simulink subsystem "bodyModel"  (R2026a)
settings: Solver=VariableStepAuto
values from neighbouring files (symbols this model uses):
  aeroParams : value not decoded    [plantParams.sldd]
  vehicleParams = 18.0    [plantParams.sldd]
libraries: matrix_library x1, vrlib x1, simulink_extras x1
settings Model: DataDictionary=plantParams.sldd  EnableAccessToBaseWorkspace=off  Creator=maxhu  LastModifiedBy=maxhu

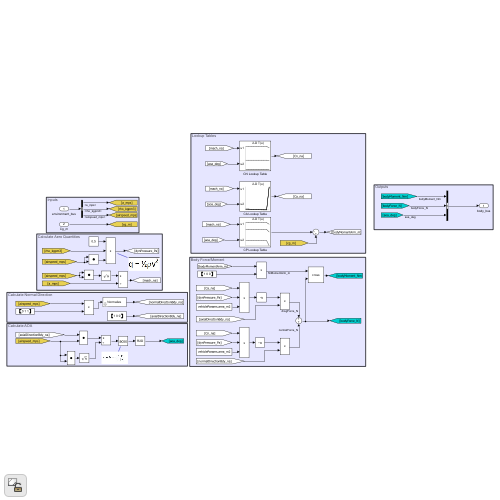
[thumbnail: Simulink's stored preview of the top-level diagram]
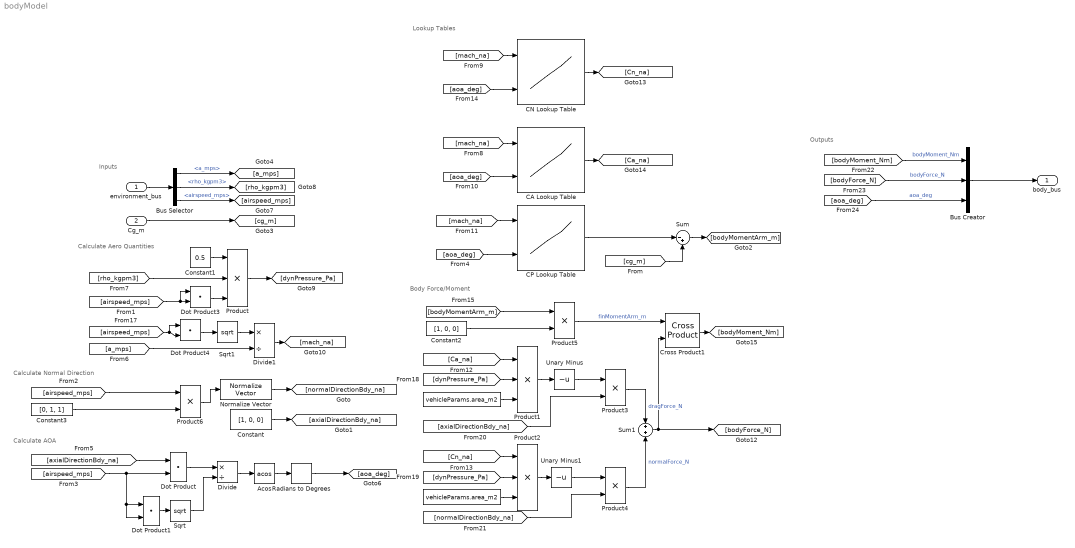
== system bodyModel ==
  note: Calculate Normal Direction
  note: Outputs
  note: Body Force/Moment
  note: Inputs
  note: Calculate Aero Quantities
  note: Calculate AOA
  note: Lookup Tables
  environment_bus : Inport
  Cg_m : Inport  Port=2
  " " : Constant  Value=vehicleParams.area_m2
  "   " : Constant  Value=vehicleParams.area_m2
  Acos : Trigonometry  Operator=acos
  Bus Creator : BusCreator  Inputs=3
  Bus Selector : BusSelector  OutputSignals=a_mps,rho_kgpm3,airspeed_mps
  CA Lookup Table : Lookup_n-D  BreakpointsForDimension1=aeroParams.machBreakpoints_na  BreakpointsForDimension2=aeroParams.aoaBreakpoints_deg  BreakpointsForDimension3=aeroParams.controlBreakpoints_deg  Table=aeroParams.CaBase_na  InternalRulePriority=Speed  RndMeth=Simplest
      settings: InputPortMap=u0,u1
  CN Lookup Table : Lookup_n-D  BreakpointsForDimension1=aeroParams.machBreakpoints_na  BreakpointsForDimension2=aeroParams.aoaBreakpoints_deg  BreakpointsForDimension3=aeroParams.controlBreakpoints_deg  Table=aeroParams.CnBase_na  InternalRulePriority=Speed  RndMeth=Simplest
      settings: InputPortMap=u0,u1
  CP Lookup Table : Lookup_n-D  BreakpointsForDimension1=aeroParams.machBreakpoints_na  BreakpointsForDimension2=aeroParams.aoaBreakpoints_deg  BreakpointsForDimension3=aeroParams.controlBreakpoints_deg  Table=aeroParams.CpBase_m  ExtrapMethod=Clip  InternalRulePriority=Speed  RndMeth=Simplest
      settings: InputPortMap=u0,u1
  Constant : Constant  Value=[1, 0, 0]
  Constant1 : Constant  Value=0.5
  Constant2 : Constant  Value=[1, 0, 0]
  Constant3 : Constant  Value=[0, 1, 1]
  Cross Product1 : matrix_library/Cross Product
  Divide : Product  Inputs=*/
  Divide1 : Product  Inputs=*/
  Dot Product{,1,3..4} (4 alike) : DotProduct  OutDataTypeStr=Inherit: Inherit via internal rule
  Normalize Vector : vrlib/Utilities/Normalize Vector  maxzero=0
  Product : Product  Inputs=3
  Product1 : Product  Inputs=3
  Product2 : Product  Inputs=3
  Product{3..6} (4 alike) : Product
  Radians to Degrees : simulink_extras/Transformations/Radians to Degrees
  Sqrt : Sqrt
  Sqrt1 : Sqrt
  Sum : Sum  Inputs=|-+
  Sum1 : Sum  Inputs=+|+
  Unary Minus : UnaryMinus
  Unary Minus1 : UnaryMinus
  body_bus : Outport
  wires:
  [axialDirectionBdy_na] -> Dot Product/1
  [airspeed_mps] -> Dot Product/2, Dot Product1/1, Dot Product1/2
  Dot Product1/1 -> Sqrt/1
  Dot Product/1 -> Divide/1
  Sqrt/1 -> Divide/2
  Divide/1 -> Acos/1
  Acos/1 -> Radians to Degrees/1
  Radians to Degrees/1 -> [aoa_deg]
  [aoa_deg] -> CN Lookup Table/2
  [aoa_deg] -> CA Lookup Table/2
  CN Lookup Table/1 -> [Cn_na]
  CA Lookup Table/1 -> [Ca_na]
  environment_bus/1 -> Bus Selector/1
  Bus Selector/3 -> [airspeed_mps]  "<airspeed_mps>"
  Bus Selector/2 -> [rho_kgpm3]  "<rho_kgpm3>"
  Bus Selector/1 -> [a_mps]  "<a_mps>"
  Product/1 -> [dynPressure_Pa]
  Constant1/1 -> Product/1
  [rho_kgpm3] -> Product/2
  [airspeed_mps] -> Dot Product3/2, Dot Product3/1
  Dot Product3/1 -> Product/3
  Divide1/1 -> [mach_na]
  [mach_na] -> CN Lookup Table/1
  [mach_na] -> CA Lookup Table/1
  [dynPressure_Pa] -> Product1/2
  Product1/1 -> Unary Minus/1
  [Ca_na] -> Product1/1
  "   "/1 -> Product1/3
  Unary Minus/1 -> Product3/1
  [axialDirectionBdy_na] -> Product3/2
  Product3/1 -> Sum1/1  "dragForce_N"
  [Cn_na] -> Product2/1
  [normalDirectionBdy_na] -> Product4/2
  Product2/1 -> Unary Minus1/1
  Unary Minus1/1 -> Product4/1
  " "/1 -> Product2/3
  [dynPressure_Pa] -> Product2/2
  Product4/1 -> Sum1/2  "normalForce_N"
  Sum1/1 -> Cross Product1/2, [bodyForce_N]
  Cross Product1/1 -> [bodyMoment_Nm]
  [aoa_deg] -> Bus Creator/3  "aoa_deg"
  [bodyForce_N] -> Bus Creator/2  "bodyForce_N"
  [bodyMoment_Nm] -> Bus Creator/1  "bodyMoment_Nm"
  Bus Creator/1 -> body_bus/1
  Sqrt1/1 -> Divide1/1
  Constant/1 -> [axialDirectionBdy_na]
  Normalize Vector/1 -> [normalDirectionBdy_na]
  Product6/1 -> Normalize Vector/1
  [airspeed_mps] -> Product6/1
  Constant3/1 -> Product6/2
  [aoa_deg] -> CP Lookup Table/2
  [mach_na] -> CP Lookup Table/1
  Sum/1 -> [bodyMomentArm_m]
  CP Lookup Table/1 -> Sum/1
  Cg_m/1 -> [cg_m]
  [cg_m] -> Sum/2
  [bodyMomentArm_m] -> Product5/1
  Constant2/1 -> Product5/2
  Product5/1 -> Cross Product1/1  "finMomentArm_m"
  [a_mps] -> Divide1/2
  Dot Product4/1 -> Sqrt1/1
  [airspeed_mps] -> Dot Product4/2, Dot Product4/1
